simulink model "AdaptiveSync_2_1"  (R2016a)
settings: Solver=ode23tb  SolverMode=SingleTasking  StartTime=0.0  StopTime=10  RelTol=1e-3
values from neighbouring files (symbols this model uses):
  A_follow = kron(eye(6),Am)+kron(L,Bm*F)    [Adaptive_Synchronization.m]
  A_sync = kron(eye(5),Am)+kron(Lnolead,Bm*F)    [Adaptive_Synchronization.m]
  x01 = [-0.5;1]    [Adaptive_Synchronization.m]
  x02 = [0.5;-1]    [Adaptive_Synchronization.m]
  x03 = [1;0.5]    [Adaptive_Synchronization.m]
  x04 = [-1;-0.5]    [Adaptive_Synchronization.m]
  x05 = [0;0]    [Adaptive_Synchronization.m]
  x0m = [0;1]    [Adaptive_Synchronization.m]
settings Model: Creator=danielvos  LastModifiedBy=danielvos
settings SolverCC: ZeroCrossAlgorithm=Adaptive
settings DebuggingCC: SFUnexpectedBacktrackingDiag=error  SFNoUnconditionalDefaultTransitionDiag=error
settings GRTTargetCC: TargetLangStandard=C99 (ISO)  GeneratePreprocessorConditionals=Use local settings
settings ConfigComp: CovMetricSettings=dwe  CovHtmlReporting=off  CovSaveCumulativeToWorkspaceVar=off  CovSaveSingleToWorkspaceVar=off  CovExternalEMLEnable=on

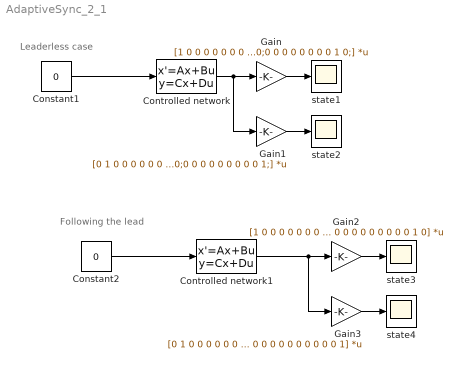
== system AdaptiveSync_2_1 ==
  note: Leaderless case
  note: Following the lead
  Constant1 : Constant  Value=0
  Constant2 : Constant  Value=0
  Controlled network : StateSpace  A=A_sync  B=zeros(10,1)  C=eye(10)  D=zeros(10,1);  X0=[x01;x02;x03;x04;x05]
  Controlled network1 : StateSpace  A=A_follow  B=zeros(12,1)  C=eye(12)  D=zeros(12,1);  X0=[x0m;x01;x02;x03;x04;x05]
  Gain : Gain  Gain=[1 0 0 0 0 0 0 0 0 0;0 0 1 0 0 0 0 0 0 0;0 0 0 0 1 0 0 0 0 0;0 0 0 0 0 0 1 0 0 0;0 0 0 0 0 0 0 0 1 0;]  Multiplication=Matrix(K*u)
  Gain1 : Gain  Gain=[0 1 0 0 0 0 0 0 0 0;0 0 0 1 0 0 0 0 0 0;0 0 0 0 0 1 0 0 0 0;0 0 0 0 0 0 0 1 0 0;0 0 0 0 0 0 0 0 0 1;]  Multiplication=Matrix(K*u)
  Gain2 : Gain  Gain=[1 0 0 0 0 0 0 0 0 0 0 0;0 0 1 0 0 0 0 0 0 0 0 0;0 0 0 0 1 0 0 0 0 0 0 0;0 0 0 0 0 0 1 0 0 0 0 0;0 0 0 0 0 0 0 0 1 0 0 0;0 0 0 0 0 0 0 0 0 0 1 0]  Multiplication=Matrix(K*u)
  Gain3 : Gain  Gain=[0 1 0 0 0 0 0 0 0 0 0 0;0 0 0 1 0 0 0 0 0 0 0 0;0 0 0 0 0 1 0 0 0 0 0 0;0 0 0 0 0 0 0 1 0 0 0 0;0 0 0 0 0 0 0 0 0 1 0 0; 0 0 0 0 0 0 0 0 0 0 0 1]  Multiplication=Matrix(K*u)
  state{1..4} (4 alike) : Scope
  wires:
  Constant1/1 -> Controlled network/1
  Controlled network/1 -> Gain1/1, Gain/1
  Constant2/1 -> Controlled network1/1
  Gain/1 -> state1/1
  Gain1/1 -> state2/1
  Controlled network1/1 -> Gain3/1, Gain2/1
  Gain3/1 -> state4/1
  Gain2/1 -> state3/1
